simulink subsystem "HEVMM"  (R2025b)
settings: Solver=VariableStepAuto  StartTime=0.0  StopTime=10.0  RelTol=1e-3
undefined symbols (not defined in the file): PlntHevMmCltchPrs, PlntHevMmEngDamp, PlntHevMmEngInertia, PlntHevMmGenGearRatio, PlntHevMmMotGearRatio
libraries: autolibsharedcoupling x5, autolibcoupling x1
settings Model: ModifiedByFormat=The MathWorks, Inc.  Creator=The MathWorks, Inc.  LastModifiedBy=The MathWorks, Inc.
settings SolverCC: MaxZcPerStep=1.0
settings DebuggingCC: UnconnectedInputMsg=warning  UnconnectedOutputMsg=warning  UnconnectedLineMsg=warning  SubsystemReferenceDiagnosticForUnitTest=warning
settings ModelReferenceCC: EnableRefExpFcnMdlSchedulingChecks=on
settings RTWCC: GPUComputeCapability=3.5  DLArmComputeVersion=19.05

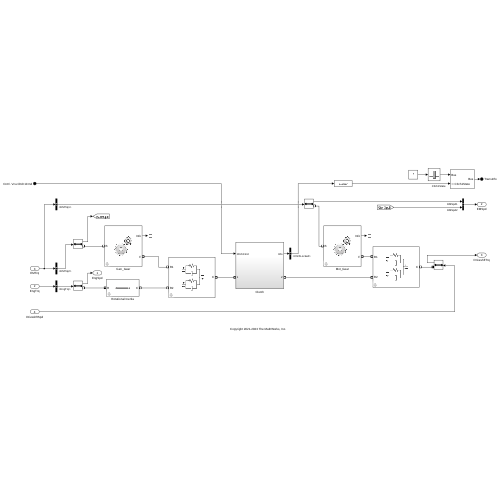
[thumbnail: Simulink's stored preview of the top-level diagram]
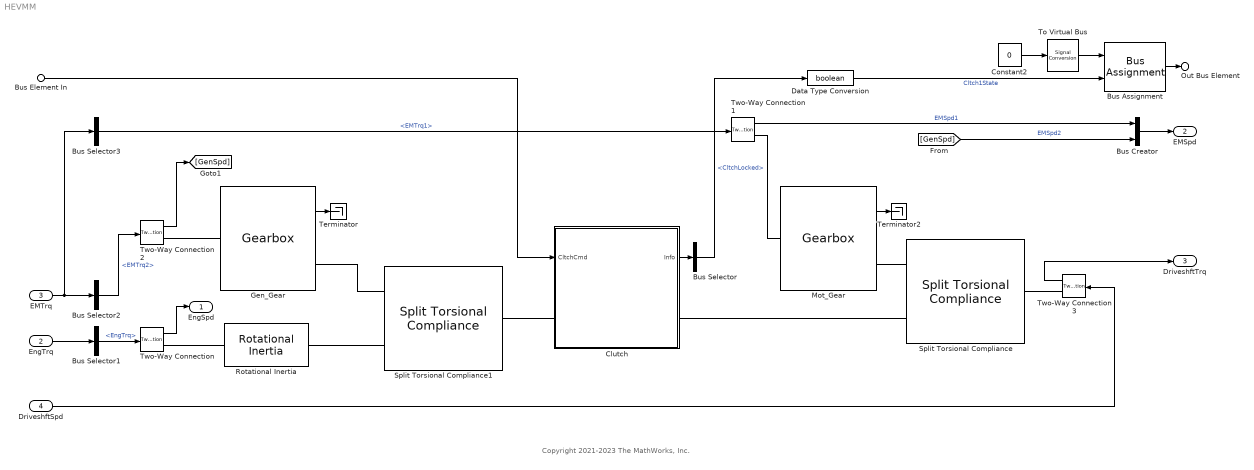
== system HEVMM ==
  note: Copyright 2021-2023 The MathWorks, Inc.
  Bus Element In : Inport  PortName=Cntrl  Element=Vcu.Cltch1Cmd
  EngTrq : Inport  Port=2
  EMTrq : Inport  Port=3
  DriveshftSpd : Inport  Port=4
  Bus Assignment : BusAssignment  AssignedSignals=Cltch1State
  Bus Creator : BusCreator  Inputs=2
  Bus Selector : BusSelector  OutputSignals=Cltch.CltchLocked
  Bus Selector1 : BusSelector  OutputSignals=EngTrq
  Bus Selector2 : BusSelector  OutputSignals=EMTrq2
  Bus Selector3 : BusSelector  OutputSignals=EMTrq1
  Clutch : Subsystem
  Constant2 : Constant  Value=0  OutDataTypeStr=Bus: TransInfoBUS  SampleTime=Inf
  Data Type Conversion : DataTypeConversion  OutDataTypeStr=boolean  SaturateOnIntegerOverflow=off  RndMeth=Floor
  Gen_Gear : autolibsharedcoupling/Gearbox  port_config=Two-way connection  input_config=Torque input - velocity output  DiffEffModelPopup=Constant  InterpMethod=Flat  dirSwitch=on  extTamb=off  N=PlntHevMmGenGearRatio  J1=PlntHevMmGenGearInInertia  J2=PlntHevMmGenGearOutInertia  b1=PlntHevMmGenGearInDamp  b2=PlntHevMmGenGearOutDamp  theta1_o=0  w1_o=PlntHevMmGenGearInitVel  eta=PlntHevMmGenGearEff  eta_tbl=reshape([0.64 0.76 0.8 0.81 0.83 0.84 0.84 0.56 0.73 0.78 0.8 0.83 0.84 0.84 0.54 0.71 0.77 0.8 0.82 0.84 0.84 0.53 0.71 0.77 0.8 0.83 0.84 0.84 0.51 0.71 0.77 0.8 0.83 0.84 0.85 0.52 0.7 0.77 0.8 0.83 0.84 0.85 0.51 0.71 0.76 0.79 0.83 0.84 0.85 0.5 0.69 0.76 0.79 0.82 0.84 0.85 0.45 0.68 0.75 0.78 0.82 0.84 0.85 0.43 0.67 0.74 0.78 0.81 0.83 0.84 0.38 0.63 0.71 0.75 0.8 0.82 0.83 0.81 0.86 0.88 0.89 0.89 0.89 0.9 0.77 0.85 0.87 0.88 0.89 0.9 0.9 0.72 0.82 0.86 0.87 0.88 0.89 0.9 0.68 0.8 0.84 0.86 0.88 0.89 0.89 0.67 0.8 0.84 0.86 0.88 0.89 0.9 0.67 0.8 0.84 0.86 0.88 0.89 0.9 0.65 0.8 0.84 0.86 0.88 0.89 0.9 0.64 0.79 0.83 0.86 0.88 0.89 0.9 0.63 0.78 0.83 0.86 0.88 0.89 0.9 0.59 0.76 0.82 0.85 0.87 0.89 0.9 0.53 0.73 0.8 0.83 0.86 0.88 0.89], 7, 11, 2)  Trq_bpts=[25, 50, 75, 100, 150, 200, 250]  omega_bpts=[52.4 78.5 105 131 157 183 209 262 314 419 524]  Temp_bpts=[290 358]  Tamb=297.15  blkID=0  aMode=1
      settings: LibrarySourceBlock=autolibcoupling/Gearbox
  Mot_Gear : autolibsharedcoupling/Gearbox  port_config=Two-way connection  input_config=Torque input - velocity output  DiffEffModelPopup=Constant  InterpMethod=Flat  dirSwitch=on  extTamb=off  N=PlntHevMmMotGearRatio  J1=PlntHevMmMotGearInInertia  J2=PlntHevMmMotGearOutInertia  b1=PlntHevMmMotGearInDamp  b2=PlntHevMmMotGearOutDamp  theta1_o=0  w1_o=PlntHevMmMotGearInitVel  eta=PlntHevMmMotGearEff  eta_tbl=reshape([0.64 0.76 0.8 0.81 0.83 0.84 0.84 0.56 0.73 0.78 0.8 0.83 0.84 0.84 0.54 0.71 0.77 0.8 0.82 0.84 0.84 0.53 0.71 0.77 0.8 0.83 0.84 0.84 0.51 0.71 0.77 0.8 0.83 0.84 0.85 0.52 0.7 0.77 0.8 0.83 0.84 0.85 0.51 0.71 0.76 0.79 0.83 0.84 0.85 0.5 0.69 0.76 0.79 0.82 0.84 0.85 0.45 0.68 0.75 0.78 0.82 0.84 0.85 0.43 0.67 0.74 0.78 0.81 0.83 0.84 0.38 0.63 0.71 0.75 0.8 0.82 0.83 0.81 0.86 0.88 0.89 0.89 0.89 0.9 0.77 0.85 0.87 0.88 0.89 0.9 0.9 0.72 0.82 0.86 0.87 0.88 0.89 0.9 0.68 0.8 0.84 0.86 0.88 0.89 0.89 0.67 0.8 0.84 0.86 0.88 0.89 0.9 0.67 0.8 0.84 0.86 0.88 0.89 0.9 0.65 0.8 0.84 0.86 0.88 0.89 0.9 0.64 0.79 0.83 0.86 0.88 0.89 0.9 0.63 0.78 0.83 0.86 0.88 0.89 0.9 0.59 0.76 0.82 0.85 0.87 0.89 0.9 0.53 0.73 0.8 0.83 0.86 0.88 0.89], 7, 11, 2)  Trq_bpts=[25, 50, 75, 100, 150, 200, 250]  omega_bpts=[52.4 78.5 105 131 157 183 209 262 314 419 524]  Temp_bpts=[290 358]  Tamb=297.15  blkID=0  aMode=1
      settings: LibrarySourceBlock=autolibcoupling/Gearbox
  Rotational Inertia : autolibsharedcoupling/Rotational Inertia  port_config=Two-way connection  extInfo=off  externJ=off  J=PlntHevMmEngInertia  b=PlntHevMmEngDamp  omega_o=PlntHevMmEngInitVel  blkID=0  aMode=1
      settings: LibrarySourceBlock=autolibcoupling/Rotational Inertia
  Split Torsional Compliance : autolibsharedcoupling/Split Torsional Compliance  port_config=Two-way connection  cplrMode=Shaft merge  extInfo=off  k1=PlntDriveshftStiff  b1=PlntDriveshftDamp  omega1_c=PlntDriveshftDampCutoffFreq  theta1_o=0  domega1_o=0  k2=PlntDriveshftStiff  b2=PlntDriveshftDamp  omega2_c=PlntDriveshftDampCutoffFreq  theta2_o=0  domega2_o=0  blkID=0  aMode=1
      settings: LibrarySourceBlock=autolibcoupling/Split Torsional Compliance
  Split Torsional Compliance1 : autolibsharedcoupling/Split Torsional Compliance  port_config=Two-way connection  cplrMode=Shaft merge  extInfo=off  k1=PlntDriveshftStiff  b1=PlntDriveshftDamp  omega1_c=PlntDriveshftDampCutoffFreq  theta1_o=0  domega1_o=0  k2=PlntDriveshftStiff  b2=PlntDriveshftDamp  omega2_c=PlntDriveshftDampCutoffFreq  theta2_o=0  domega2_o=0  blkID=0  aMode=1
      settings: LibrarySourceBlock=autolibcoupling/Split Torsional Compliance
  Terminator : Terminator
  Terminator2 : Terminator
  To Virtual Bus : SignalConversion  ConversionOutput=Virtual bus  OverrideOpt=off
  Two-Way Connection{,1..3} (4 alike) : TwoWayConnection
  EngSpd : Outport  VectorParamsAs1DForOutWhenUnconnected=off  BusOutputAsStruct=on
  EMSpd : Outport  Port=2  VectorParamsAs1DForOutWhenUnconnected=off  BusOutputAsStruct=on
  DriveshftTrq : Outport  Port=3  VectorParamsAs1DForOutWhenUnconnected=off
  Out Bus Element : Outport  Port=4  PortName=TransInfo
  wires:
  Bus Selector/1 -> Data Type Conversion/1  "<CltchLocked>"
  Mot_Gear/1 -> Terminator2/1
  Two-Way Connection1/1 -> Bus Creator/1  "EMSpd1"
  Clutch/1(Info) -> Bus Selector/1
  EMTrq/1 -> Bus Selector2/1, Bus Selector3/1
  EngTrq/1 -> Bus Selector1/1
  Bus Element In/1 -> Clutch/1(CltchCmd)
  Gen_Gear/1 -> Terminator/1
  Bus Selector3/1 -> Two-Way Connection1/1  "<EMTrq1>"
  Two-Way Connection/1 -> EngSpd/1
  Bus Creator/1 -> EMSpd/1
  [GenSpd] -> Bus Creator/2  "EMSpd2"
  DriveshftSpd/1 -> Two-Way Connection3/1
  Two-Way Connection3/1 -> DriveshftTrq/1
  Bus Selector2/1 -> Two-Way Connection2/1  "<EMTrq2>"
  Two-Way Connection2/1 -> [GenSpd]
  Bus Assignment/1 -> Out Bus Element/1
  Data Type Conversion/1 -> Bus Assignment/2  "Cltch1State"
  Constant2/1 -> To Virtual Bus/1
  To Virtual Bus/1 -> Bus Assignment/1
  Bus Selector1/1 -> Two-Way Connection/1  "<EngTrq>"
  connections:
  Two-Way Connection1/RConn1 -- Mot_Gear/LConn1
  Mot_Gear/RConn1 -- Split Torsional Compliance/LConn1
  Clutch/RConn1 -- Split Torsional Compliance/LConn2
  Two-Way Connection3/RConn1 -- Split Torsional Compliance/RConn1
  Two-Way Connection2/RConn1 -- Gen_Gear/LConn1
  Split Torsional Compliance1/RConn1 -- Clutch/LConn1
  Gen_Gear/RConn1 -- Split Torsional Compliance1/LConn1
  Rotational Inertia/RConn1 -- Split Torsional Compliance1/LConn2
  Rotational Inertia/LConn1 -- Two-Way Connection/RConn1

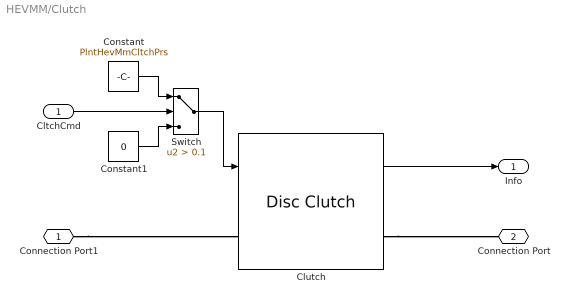
== system HEVMM/Clutch ==
  CltchCmd : Inport
  Clutch : autolibcoupling/Disc Clutch  port_config=Two-way connection  Reff=PlntCltch1Radius  Ndisk=PlntCltch1NumDisk  Aeff=PlntCltch1AppPrsArea  Peng=PlntCltch1EngdPrs  Jin=PlntHevMmCltchInInertia  Jout=PlntCltch1OutInertia  muk=PlntCltch1KinFric  mus=PlntCltch1StatFric  bin=PlntCltch1InDamp  bout=PlntCltch1OutDamp  win_o=PlntCltch1InitInVel  wout_o=PlntCltch1InitOutVel  tauC=PlntHevMmCltchTimeCnst  InitiallyLocked=off  maxAbsSpd=3000  blkID=1
  Constant : Constant  Value=PlntHevMmCltchPrs  SampleTime=-1
  Constant1 : Constant  Value=0
  Switch : Switch  Criteria=u2 > Threshold  Threshold=0.1  SaturateOnIntegerOverflow=off  InputSameDT=off
  Connection Port1 : PMIOPort  Side=Left
  Connection Port : PMIOPort  Port=2  Side=Right
  Info : Outport  VectorParamsAs1DForOutWhenUnconnected=off
  wires:
  Switch/1 -> Clutch/1
  Clutch/1 -> Info/1
  Constant1/1 -> Switch/3
  CltchCmd/1 -> Switch/2
  Constant/1 -> Switch/1
  connections:
  Connection Port1/RConn1 -- Clutch/LConn1
  Clutch/RConn1 -- Connection Port/RConn1
